simulink library "models"  (Simulink 7.2)
settings: Solver=ode45  SolverMode=SingleTasking  StartTime=0.0  StopTime=10.0  RelTol=1e-3
undefined symbols (not defined in the file or in its folder): actuator_T2_lib, aero, Aero, aero_lib, aftfuel, aftfuel_pos, Am, atmos, b, bias, Bm, Cbar, cg_pos0, cg_shift_gear, constants, DamageModels, Ed_trim_IC, engl_ang, engl_pos, engr_ang, engr_pos, fwdfuel, fwdfuel_pos, GTM_T2, hd_trim_IC, in_tadapton_forced, Inertia0, Inertia_shift_gear, latlonh_IC, MACH_U_nom_IC, Nd_trim_IC, pqr_trim_IC, quat_trim_IC, ref_cg, S, SENSOR, SERVO, symmetric_aero_on, trac_params, use_wind_meas_sim, vehicle_params, w0, xm0
libraries: simulink_need_slupdate x56, models x11, aeroutilslib x6, utility_lib x5, GTM_aerolib x4, model_lib x4, Polyval_lib x3, simulink x2, enginelib x2, engine_T2_lib x1
(part 1 of 4)
settings Model: Creator=E183308  LastModifiedBy=E183308

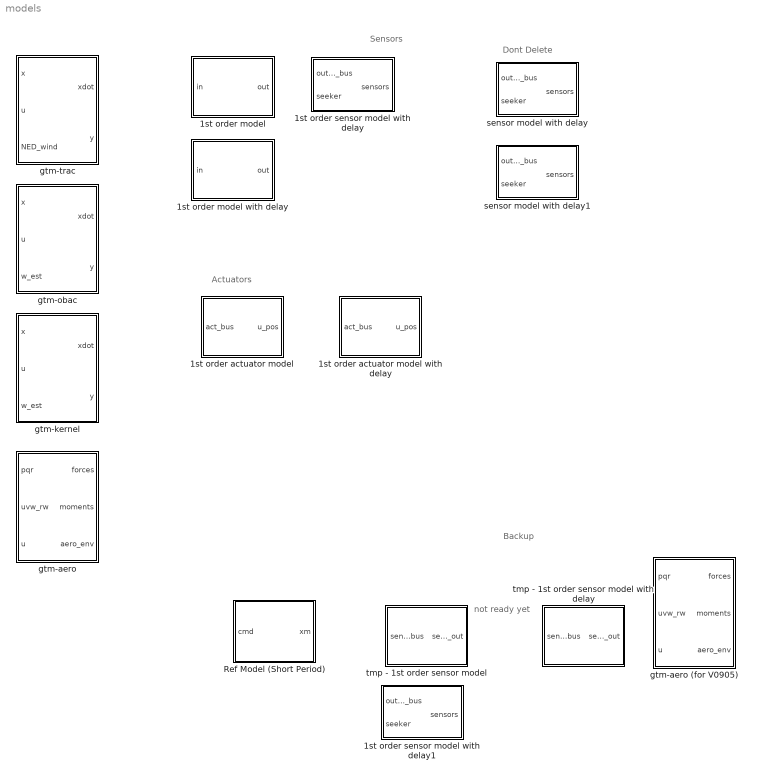
== system models ==
  note: Backup
  note: not ready yet
  note: Actuators
  note: Sensors
  note: Dont Delete
  1st order actuator model : Subsystem
  1st order actuator model with delay : Subsystem
  1st order model : Subsystem  mask{sens_idx=0}
      mask prompts: sens_idx "Indices"
  1st order model with delay : Subsystem  mask{sens_idx=0}
      mask prompts: sens_idx "Indices"
  1st order sensor model with delay : Subsystem
  1st order sensor model with delay1 : Subsystem
  Ref Model (Short Period) : Subsystem
  gtm-aero : Subsystem  mask{aero_params=aero}
      mask prompts: aero_params "aero params"
      mask init:
      | paramnames = fieldnames(aero_params);
      | for i=1:length(paramnames)
      | 	eval([paramnames{i} '= aero_params.' paramnames{i} ';']);
      | end
  gtm-aero (for V0905) : Subsystem  mask{aero_params=aero}
      mask prompts: aero_params "aero params"
      mask init:
      | paramnames = fieldnames(aero_params);
      | for i=1:length(paramnames)
      | 	eval([paramnames{i} '= aero_params.' paramnames{i} ';']);
      | end
  gtm-kernel : Subsystem  mask{vehicle_params=vehicle_params}
      mask prompts: vehicle_params "vehicle params"
      mask init:
      | paramnames = fieldnames(vehicle_params);
      | for i=1:length(paramnames)
      | 	eval([paramnames{i} '= vehicle_params.' paramnames{i} ';']);
      | end
  gtm-obac : Subsystem
  gtm-trac : Subsystem  mask{vehicle_params=trac_params}
      mask prompts: vehicle_params "vehicle params"
  sensor model with delay : Subsystem
  sensor model with delay1 : Subsystem
  tmp - 1st order sensor model : Subsystem
  tmp - 1st order sensor model with delay : Subsystem

== system models/1st order actuator model ==
  note: VARIABLE RATE LIMIT SERVO MODEL
      | (1st order)
  act_bus : Inport  OutDataType=sfix(16)  OutScaling=2^0
  Bus Selector1 : BusSelector  OutputSignals=effector_limits.u_ulim,effector_limits.u_llim,effector_limits.u_urlim,effector_limits.u_lrlim,u_cmd
  Enforce lower limit : MinMax  Function=max  Inputs=2  OutDataType=sfix(16)  OutScaling=2^-10  OutDataTypeStr=Inherit: Inherit via back propagation  ZeroCross=off
  Enforce lower limit1 : MinMax  Function=max  Inputs=2  OutDataType=sfix(16)  OutScaling=2^-10  OutDataTypeStr=Inherit: Inherit via back propagation  ZeroCross=off
  Enforce upper limit : MinMax  Inputs=2  OutDataType=sfix(16)  OutScaling=2^-10  OutDataTypeStr=Inherit: Inherit via back propagation  ZeroCross=off
  Enforce upper limit1 : MinMax  Inputs=2  OutDataType=sfix(16)  OutScaling=2^-10  OutDataTypeStr=Inherit: Inherit via back propagation  ZeroCross=off
  Sum : Sum  Inputs=|+-  OutDataType=sfix(16)  OutScaling=2^0  SaturateOnIntegerOverflow=on  InputSameDT=on  OutDataTypeStr=Inherit: Same as first input
  Sum1 : Sum  Inputs=|++  OutDataType=sfix(16)  OutScaling=2^0  SaturateOnIntegerOverflow=on  InputSameDT=on  OutDataTypeStr=Inherit: Same as first input
  Sum2 : Sum  Orientation=left  Inputs=-+|  OutDataType=sfix(16)  OutScaling=2^0  SaturateOnIntegerOverflow=on  InputSameDT=on  OutDataTypeStr=Inherit: Same as first input
  W : Gain  Gain=SERVO.w  ParameterDataType=sfix(16)  ParameterScaling=2^0  OutDataType=sfix(16)  OutScaling=2^0  SaturateOnIntegerOverflow=on  OutDataTypeStr=Inherit: Same as input  ParamDataTypeStr=Inherit: Same as input
  anti-windup gain : Gain  Orientation=left  Gain=SERVO.pos_Kaw  ParameterDataType=sfix(16)  ParameterScaling=2^0  OutDataType=sfix(16)  OutScaling=2^0
  pos integrator : Integrator  InitialCondition=SERVO.x0
  u_pos : Outport  OutDataType=sfix(16)  OutScaling=2^0
  wires:
  Bus Selector1/4 -> Enforce lower limit1/1  "<u_lrlim>"
  Bus Selector1/1 -> Enforce upper limit/1  "<u_ulim>"
  act_bus/1 -> Bus Selector1/1
  Enforce upper limit/1 -> Sum2/2, Sum/2, u_pos/1
  Enforce lower limit/1 -> Enforce upper limit/2
  pos integrator/1 -> Sum2/1, Enforce lower limit/2
  Sum2/1 -> anti-windup gain/1
  anti-windup gain/1 -> Sum1/2
  Sum1/1 -> pos integrator/1
  Sum/1 -> W/1
  Bus Selector1/5 -> Sum/1  "<u_cmd>"
  Bus Selector1/2 -> Enforce lower limit/1  "<u_llim>"
  Bus Selector1/3 -> Enforce upper limit1/1  "<u_urlim>"
  W/1 -> Enforce lower limit1/2
  Enforce lower limit1/1 -> Enforce upper limit1/2
  Enforce upper limit1/1 -> Sum1/1

== system models/1st order actuator model with delay ==
  note: VARIABLE RATE LIMIT SERVO MODEL
      | (1st order with delay)
  act_bus : Inport  OutDataType=sfix(16)  OutScaling=2^0
  1st order actuator model : models/1st order actuator model  SystemSampleTime=-1
  Transport Delay : TransportDelay  DelayTime=SERVO.delay  InitialOutput=SERVO.x0
  u_pos : Outport  OutDataType=sfix(16)  OutScaling=2^0
  wires:
  act_bus/1 -> 1st order actuator model/1
  1st order actuator model/1 -> Transport Delay/1
  Transport Delay/1 -> u_pos/1

== system models/1st order model ==
  note: 1st ORDER LIMIT MODEL
  in : Inport  OutDataType=sfix(16)  OutScaling=2^0
  Constant : Constant  Value=SENSOR.ulim(sens_idx)  OutDataType=sfix(16)  OutScaling=2^0
  Constant1 : Constant  Value=SENSOR.llim(sens_idx)  OutDataType=sfix(16)  OutScaling=2^0
  Enforce lower limit : MinMax  Function=max  Inputs=2  OutDataType=sfix(16)  OutScaling=2^-10  OutDataTypeStr=Inherit: Inherit via back propagation  ZeroCross=off
  Enforce upper limit : MinMax  Inputs=2  OutDataType=sfix(16)  OutScaling=2^-10  OutDataTypeStr=Inherit: Inherit via back propagation  ZeroCross=off
  Sum : Sum  Inputs=|+-  OutDataType=sfix(16)  OutScaling=2^0  SaturateOnIntegerOverflow=on  InputSameDT=on  OutDataTypeStr=Inherit: Same as first input
  W : Gain  Gain=SENSOR.w(sens_idx)  ParameterDataType=sfix(16)  ParameterScaling=2^0  OutDataType=sfix(16)  OutScaling=2^0  SaturateOnIntegerOverflow=on  OutDataTypeStr=Inherit: Same as input  ParamDataTypeStr=Inherit: Same as input
  integrator : Integrator  InitialCondition=SENSOR.x0(sens_idx)
  out : Outport  OutDataType=sfix(16)  OutScaling=2^0
  wires:
  Constant1/1 -> Enforce lower limit/1
  Sum/1 -> W/1
  integrator/1 -> Enforce lower limit/2
  Enforce lower limit/1 -> Enforce upper limit/2
  Enforce upper limit/1 -> out/1, Sum/2
  Constant/1 -> Enforce upper limit/1
  W/1 -> integrator/1
  in/1 -> Sum/1

== system models/1st order model with delay ==
  note: 1st ORDER LIMIT MODEL WITH DELAY
  in : Inport  OutDataType=sfix(16)  OutScaling=2^0
  Constant : Constant  Value=SENSOR.ulim(sens_idx)  OutDataType=sfix(16)  OutScaling=2^0
  Constant1 : Constant  Value=SENSOR.llim(sens_idx)  OutDataType=sfix(16)  OutScaling=2^0
  Enforce lower limit : MinMax  Function=max  Inputs=2  OutDataType=sfix(16)  OutScaling=2^-10  OutDataTypeStr=Inherit: Inherit via back propagation  ZeroCross=off
  Enforce upper limit : MinMax  Inputs=2  OutDataType=sfix(16)  OutScaling=2^-10  OutDataTypeStr=Inherit: Inherit via back propagation  ZeroCross=off
  Sum : Sum  Inputs=|+-  OutDataType=sfix(16)  OutScaling=2^0  SaturateOnIntegerOverflow=on  InputSameDT=on  OutDataTypeStr=Inherit: Same as first input
  W : Gain  Gain=SENSOR.w(sens_idx)  ParameterDataType=sfix(16)  ParameterScaling=2^0  OutDataType=sfix(16)  OutScaling=2^0  SaturateOnIntegerOverflow=on  OutDataTypeStr=Inherit: Same as input  ParamDataTypeStr=Inherit: Same as input
  delay : TransportDelay  DelayTime=SENSOR.delay  InitialOutput=SENSOR.x0(sens_idx)
  integrator : Integrator  InitialCondition=SENSOR.x0(sens_idx)
  out : Outport  OutDataType=sfix(16)  OutScaling=2^0
  wires:
  in/1 -> Sum/1
  W/1 -> integrator/1
  Constant/1 -> Enforce upper limit/1
  Enforce upper limit/1 -> Sum/2, delay/1
  Enforce lower limit/1 -> Enforce upper limit/2
  integrator/1 -> Enforce lower limit/2
  Sum/1 -> W/1
  Constant1/1 -> Enforce lower limit/1
  delay/1 -> out/1

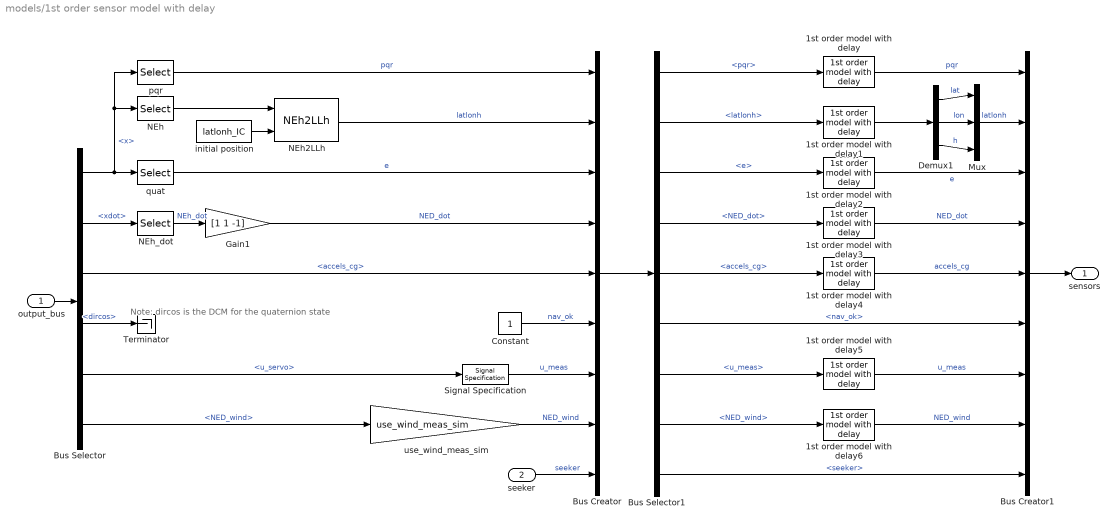
== system models/1st order sensor model with delay ==
  note: Note: dircos is the DCM
      | for the quaternion state
  output_bus : Inport  OutDataType=sfix(16)  OutScaling=2^0
  seeker : Inport  Port=2  OutDataType=sfix(16)  OutScaling=2^0
  1st order model with delay : models/1st order model with delay  SystemSampleTime=-1  sens_idx=SENSOR.pqr_idx
  1st order model with delay1 : models/1st order model with delay  SystemSampleTime=-1  sens_idx=SENSOR.latlonh_idx
  1st order model with delay2 : models/1st order model with delay  SystemSampleTime=-1  sens_idx=SENSOR.quat_idx
  1st order model with delay3 : models/1st order model with delay  SystemSampleTime=-1  sens_idx=SENSOR.NEDdot_idx
  1st order model with delay4 : models/1st order model with delay  SystemSampleTime=-1  sens_idx=SENSOR.accels_cg_idx
  1st order model with delay5 : models/1st order model with delay  SystemSampleTime=-1  sens_idx=SENSOR.umeas_idx
  1st order model with delay6 : models/1st order model with delay  SystemSampleTime=-1  sens_idx=SENSOR.NED_wind_idx
  Bus Creator : BusCreator  Inputs=9
  Bus Creator1 : BusCreator  Inputs=9
  Bus Selector : BusSelector  OutputSignals=x,xdot,y.accels_cg,y.dircos,u_servo,NED_wind
  Bus Selector1 : BusSelector  OutputSignals=pqr,latlonh,e,NED_dot,accels_cg,nav_ok,u_meas,NED_wind,seeker
  Constant : Constant  OutDataType=sfix(16)  OutScaling=2^0
  Demux1 : Demux  Outputs=3
  Gain1 : Gain  Gain=[1 1 -1]  ParameterDataType=sfix(16)  ParameterScaling=2^0  OutDataType=sfix(16)  OutScaling=2^0  SaturateOnIntegerOverflow=on  OutDataTypeStr=Inherit: Same as input  ParamDataTypeStr=Inherit: Same as input
  Mux : Mux  Inputs=3
  NEh : Selector  InputPortWidth=MACH.num_x  IndexOptions=Index vector (dialog)  Indices=MACH.NEh_idx  OutputSizes=1
  NEh2LLh : utility_lib/NEh2LLh  SystemSampleTime=-1
  NEh_dot : Selector  InputPortWidth=MACH.num_x  IndexOptions=Index vector (dialog)  Indices=MACH.NEh_idx  OutputSizes=1
  Signal Specification : SignalSpecification  OutDataType=sfix(16)  OutScaling=2^0
  Terminator : Terminator
  initial position : Constant  Value=latlonh_IC  OutDataType=sfix(16)  OutScaling=2^0
  pqr : Selector  InputPortWidth=MACH.num_x  IndexOptions=Index vector (dialog)  Indices=MACH.pqr_idx  OutputSizes=1
  quat : Selector  InputPortWidth=MACH.num_x  IndexOptions=Index vector (dialog)  Indices=MACH.quat_idx  OutputSizes=1
  use_wind_meas_sim : Gain  Gain=use_wind_meas_sim  ParameterDataType=sfix(16)  ParameterScaling=2^0  OutDataType=sfix(16)  OutScaling=2^0  SaturateOnIntegerOverflow=on  OutDataTypeStr=Inherit: Same as input  ParamDataTypeStr=Inherit: Same as input
  sensors : Outport  OutDataType=sfix(16)  OutScaling=2^0
  wires:
  1st order model with delay4/1 -> Bus Creator1/5  "accels_cg"
  1st order model with delay3/1 -> Bus Creator1/4  "NED_dot"
  1st order model with delay2/1 -> Bus Creator1/3  "e"
  1st order model with delay1/1 -> Demux1/1
  1st order model with delay6/1 -> Bus Creator1/8  "NED_wind"
  Bus Selector1/8 -> 1st order model with delay6/1  "<NED_wind>"
  1st order model with delay5/1 -> Bus Creator1/7  "u_meas"
  Bus Selector1/7 -> 1st order model with delay5/1  "<u_meas>"
  Bus Selector1/5 -> 1st order model with delay4/1  "<accels_cg>"
  Bus Selector1/4 -> 1st order model with delay3/1  "<NED_dot>"
  Bus Selector1/3 -> 1st order model with delay2/1  "<e>"
  Bus Selector1/2 -> 1st order model with delay1/1  "<latlonh>"
  Bus Selector1/1 -> 1st order model with delay/1  "<pqr>"
  Bus Selector1/9 -> Bus Creator1/9  "<seeker>"
  1st order model with delay/1 -> Bus Creator1/1  "pqr"
  Bus Creator/1 -> Bus Selector1/1
  Mux/1 -> Bus Creator1/2  "latlonh"
  Demux1/3 -> Mux/3  "h"
  Demux1/2 -> Mux/2  "lon"
  Demux1/1 -> Mux/1  "lat"
  Bus Creator1/1 -> sensors/1
  Signal Specification/1 -> Bus Creator/7  "u_meas"
  Bus Selector/5 -> Signal Specification/1  "<u_servo>"
  use_wind_meas_sim/1 -> Bus Creator/8  "NED_wind"
  Gain1/1 -> Bus Creator/4  "NED_dot"
  NEh2LLh/1 -> Bus Creator/2  "latlonh"
  pqr/1 -> Bus Creator/1  "pqr"
  NEh_dot/1 -> Gain1/1  "NEh_dot"
  Bus Selector/2 -> NEh_dot/1  "<xdot>"
  quat/1 -> Bus Creator/3  "e"
  initial position/1 -> NEh2LLh/2
  Constant/1 -> Bus Creator/6  "nav_ok"
  NEh/1 -> NEh2LLh/1
  output_bus/1 -> Bus Selector/1
  Bus Selector/6 -> use_wind_meas_sim/1  "<NED_wind>"
  seeker/1 -> Bus Creator/9  "seeker"
  Bus Selector/1 -> quat/1, NEh/1, pqr/1  "<x>"
  Bus Selector/3 -> Bus Creator/5  "<accels_cg>"
  Bus Selector/4 -> Terminator/1  "<dircos>"
  Bus Selector1/6 -> Bus Creator1/6  "<nav_ok>"

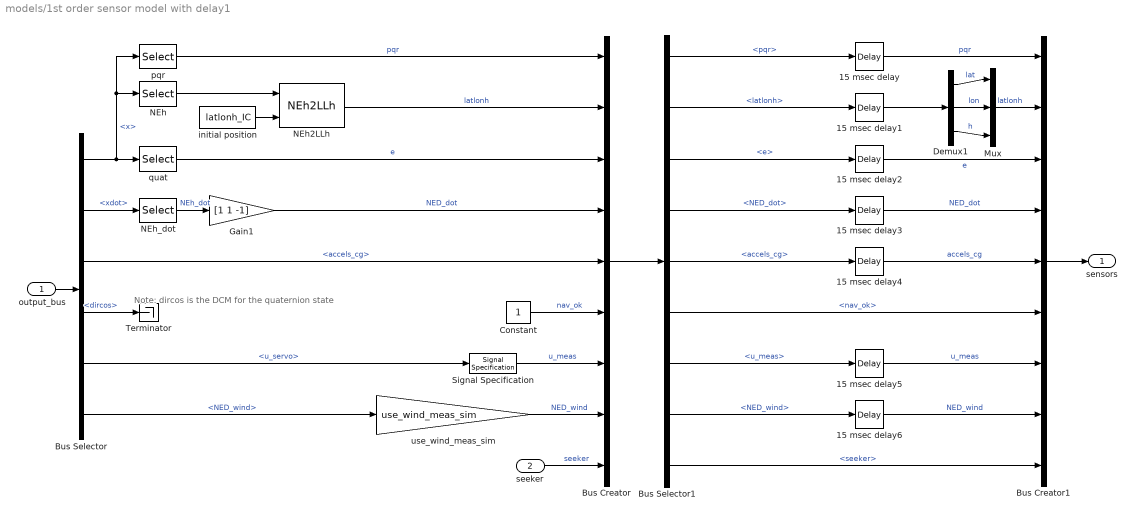
== system models/1st order sensor model with delay1 ==
  note: Note: dircos is the DCM
      | for the quaternion state
  output_bus : Inport  OutDataType=sfix(16)  OutScaling=2^0
  seeker : Inport  Port=2  OutDataType=sfix(16)  OutScaling=2^0
  15 msec delay : TransportDelay  DelayTime=15e-3  InitialOutput=pqr_trim_IC
  15 msec delay1 : TransportDelay  DelayTime=15e-3  InitialOutput=latlonh_IC
  15 msec delay2 : TransportDelay  DelayTime=15e-3  InitialOutput=quat_trim_IC
  15 msec delay3 : TransportDelay  DelayTime=15e-3  InitialOutput=[Nd_trim_IC Ed_trim_IC -hd_trim_IC]
  15 msec delay4 : TransportDelay  DelayTime=15e-3  InitialOutput=[0 0 0]'
  15 msec delay5 : TransportDelay  DelayTime=15e-3  InitialOutput=MACH_U_nom_IC
  15 msec delay6 : TransportDelay  DelayTime=15e-3  InitialOutput=[0 0 0]'
  Bus Creator : BusCreator  Inputs=9
  Bus Creator1 : BusCreator  Inputs=9
  Bus Selector : BusSelector  OutputSignals=x,xdot,y.accels_cg,y.dircos,u_servo,NED_wind
  Bus Selector1 : BusSelector  OutputSignals=pqr,latlonh,e,NED_dot,accels_cg,nav_ok,u_meas,NED_wind,seeker
  Constant : Constant  OutDataType=sfix(16)  OutScaling=2^0
  Demux1 : Demux  Outputs=3
  Gain1 : Gain  Gain=[1 1 -1]  ParameterDataType=sfix(16)  ParameterScaling=2^0  OutDataType=sfix(16)  OutScaling=2^0  SaturateOnIntegerOverflow=on  OutDataTypeStr=Inherit: Same as input  ParamDataTypeStr=Inherit: Same as input
  Mux : Mux  Inputs=3
  NEh : Selector  InputPortWidth=MACH.num_x  IndexOptions=Index vector (dialog)  Indices=MACH.NEh_idx  OutputSizes=1
  NEh2LLh : utility_lib/NEh2LLh  SystemSampleTime=-1
  NEh_dot : Selector  InputPortWidth=MACH.num_x  IndexOptions=Index vector (dialog)  Indices=MACH.NEh_idx  OutputSizes=1
  Signal Specification : SignalSpecification  OutDataType=sfix(16)  OutScaling=2^0
  Terminator : Terminator
  initial position : Constant  Value=latlonh_IC  OutDataType=sfix(16)  OutScaling=2^0
  pqr : Selector  InputPortWidth=MACH.num_x  IndexOptions=Index vector (dialog)  Indices=MACH.pqr_idx  OutputSizes=1
  quat : Selector  InputPortWidth=MACH.num_x  IndexOptions=Index vector (dialog)  Indices=MACH.quat_idx  OutputSizes=1
  use_wind_meas_sim : Gain  Gain=use_wind_meas_sim  ParameterDataType=sfix(16)  ParameterScaling=2^0  OutDataType=sfix(16)  OutScaling=2^0  SaturateOnIntegerOverflow=on  OutDataTypeStr=Inherit: Same as input  ParamDataTypeStr=Inherit: Same as input
  sensors : Outport  OutDataType=sfix(16)  OutScaling=2^0
  wires:
  Bus Selector1/6 -> Bus Creator1/6  "<nav_ok>"
  Bus Selector/4 -> Terminator/1  "<dircos>"
  Bus Selector/3 -> Bus Creator/5  "<accels_cg>"
  Bus Selector/1 -> pqr/1, NEh/1, quat/1  "<x>"
  seeker/1 -> Bus Creator/9  "seeker"
  Bus Selector/6 -> use_wind_meas_sim/1  "<NED_wind>"
  output_bus/1 -> Bus Selector/1
  NEh/1 -> NEh2LLh/1
  Constant/1 -> Bus Creator/6  "nav_ok"
  initial position/1 -> NEh2LLh/2
  quat/1 -> Bus Creator/3  "e"
  Bus Selector/2 -> NEh_dot/1  "<xdot>"
  NEh_dot/1 -> Gain1/1  "NEh_dot"
  pqr/1 -> Bus Creator/1  "pqr"
  NEh2LLh/1 -> Bus Creator/2  "latlonh"
  Gain1/1 -> Bus Creator/4  "NED_dot"
  use_wind_meas_sim/1 -> Bus Creator/8  "NED_wind"
  Bus Selector/5 -> Signal Specification/1  "<u_servo>"
  Signal Specification/1 -> Bus Creator/7  "u_meas"
  Bus Creator1/1 -> sensors/1
  Demux1/1 -> Mux/1  "lat"
  Demux1/2 -> Mux/2  "lon"
  Demux1/3 -> Mux/3  "h"
  Mux/1 -> Bus Creator1/2  "latlonh"
  Bus Creator/1 -> Bus Selector1/1
  15 msec delay/1 -> Bus Creator1/1  "pqr"
  Bus Selector1/9 -> Bus Creator1/9  "<seeker>"
  Bus Selector1/1 -> 15 msec delay/1  "<pqr>"
  Bus Selector1/2 -> 15 msec delay1/1  "<latlonh>"
  Bus Selector1/3 -> 15 msec delay2/1  "<e>"
  Bus Selector1/4 -> 15 msec delay3/1  "<NED_dot>"
  Bus Selector1/5 -> 15 msec delay4/1  "<accels_cg>"
  Bus Selector1/7 -> 15 msec delay5/1  "<u_meas>"
  15 msec delay5/1 -> Bus Creator1/7  "u_meas"
  Bus Selector1/8 -> 15 msec delay6/1  "<NED_wind>"
  15 msec delay6/1 -> Bus Creator1/8  "NED_wind"
  15 msec delay1/1 -> Demux1/1
  15 msec delay2/1 -> Bus Creator1/3  "e"
  15 msec delay3/1 -> Bus Creator1/4  "NED_dot"
  15 msec delay4/1 -> Bus Creator1/5  "accels_cg"

== system models/Ref Model (Short Period) ==
  cmd : Inport  OutDataType=sfix(16)  OutScaling=2^0
  Am : Gain  Orientation=left  Gain=Am  Multiplication=Matrix(K*u)  ParameterDataType=sfix(16)  ParameterScaling=2^0  OutDataType=sfix(16)  OutScaling=2^0
  Bm : Gain  Gain=Bm  Multiplication=Matrix(K*u)  ParameterDataType=sfix(16)  ParameterScaling=2^0  OutDataType=sfix(16)  OutScaling=2^0
  Clock : Clock
      settings: Decimation=10
  Compare To Constant : simulink/Logic and Bit Operations/Compare To Constant  SystemSampleTime=-1  relop=>=  const=in_tadapton_forced  LogicOutDataTypeMode=boolean  ZeroCross=off
  Constant : Constant  Value=[0 0 0]  OutDataType=sfix(16)  OutScaling=2^0
  Constant1 : Constant  Value="[0.0215    0.0052    0.0041]"  OutDataType=sfix(16)  OutScaling=2^0
  Gain : Gain  Gain=180/pi  ParameterDataType=sfix(16)  ParameterScaling=2^0  OutDataType=sfix(16)  OutScaling=2^0
  Gain1 : Gain  Gain=180/pi  ParameterDataType=sfix(16)  ParameterScaling=2^0  OutDataType=sfix(16)  OutScaling=2^0
  Gain2 : Gain  Gain=180/pi  ParameterDataType=sfix(16)  ParameterScaling=2^0  OutDataType=sfix(16)  OutScaling=2^0
  Integrator : Integrator  ExternalReset=rising  InitialConditionSource=external  InitialCondition=xm0
  Sum2 : Sum  Inputs=|++  OutDataType=sfix(16)  OutScaling=2^0
  Switch : Switch  Threshold=in_tadapton_forced  OutDataType=sfix(16)  OutScaling=2^0
  alpha (deg) : Scope
      settings: SaveName=ScopeData22
  alpham : Selector  InputPortWidth=3  IndexOptions=Index vector (dialog)  Indices=3  OutputSizes=1
  qcmd (deg/s) : Scope
      settings: YMin=-1  YMax=1  SaveName=ScopeData5
  qm : Selector  InputPortWidth=3  IndexOptions=Index vector (dialog)  Indices=2  OutputSizes=1
  qm (deg/s) : Scope
      settings: SaveName=ScopeData3
  qm1 : Selector  InputPortWidth=3  IndexOptions=Index vector (dialog)  Indices=1  OutputSizes=1
  xcm : Scope
      settings: SaveName=ScopeData9
  xm : Outport  OutDataType=sfix(16)  OutScaling=2^0
  wires:
  cmd/1 -> Bm/1, Gain2/1
  Integrator/1 -> Am/1, xm/1, qm1/1, qm/1, alpham/1
  Am/1 -> Sum2/2
  Sum2/1 -> Integrator/1
  Bm/1 -> Sum2/1
  qm/1 -> Gain/1
  alpham/1 -> Gain1/1
  Gain/1 -> qm (deg/s)/1
  Gain1/1 -> alpha (deg)/1
  Gain2/1 -> qcmd (deg/s)/1
  qm1/1 -> xcm/1
  Switch/1 -> Integrator/3
  Constant1/1 -> Switch/1
  Constant/1 -> Switch/3
  Clock/1 -> Switch/2, Compare To Constant/1
  Compare To Constant/1 -> Integrator/2

== system models/gtm-aero ==
  pqr : Inport  OutDataType=sfix(16)  OutScaling=2^0
  uvw_rw : Inport  Port=2  OutDataType=sfix(16)  OutScaling=2^0
  u : Inport  Port=3  OutDataType=sfix(16)  OutScaling=2^0
  A/C parameters : Subsystem  AncestorBlock=acparams_lib/A//C parameters
  Aero_GTM_T2 : Subsystem  AncestorBlock=aero_lib/GTM_T2
  AuxVars_Reduced : Subsystem
  Bus Selector4 : BusSelector  OutputSignals=atmos_env.sos,atmos_env.rho,atmos_env.h,atmos_env.P,atmos_env.T
  Demux : Demux  Outputs=[3 3]
  GTM_T2_MACH : engine_T2_lib/GTM_T2_MACH  SystemSampleTime=-1
  Goto Tag Visibility : GotoTagVisibility  GotoTag=AC_Params
  Sum : Sum  OutDataType=sfix(16)  OutScaling=2^0
  Terminator : Terminator
  aero surf ganging : Subsystem
  get aero environment : model_lib/get aero environment  SystemSampleTime=-1
  forces : Outport  OutDataType=sfix(16)  OutScaling=2^0
  moments : Outport  Port=2  OutDataType=sfix(16)  OutScaling=2^0
  aero_env : Outport  Port=3  OutDataType=sfix(16)  OutScaling=2^0
  tag scope: AC_Params=scoped
  wires:
  u/1 -> aero surf ganging/1(u)
  uvw_rw/1 -> get aero environment/1
  pqr/1 -> AuxVars_Reduced/1(pqr)
  get aero environment/1 -> aero_env/1, AuxVars_Reduced/2(aero_env)
  Bus Selector4/1 -> get aero environment/2  "<sos>"
  Bus Selector4/2 -> get aero environment/3  "<rho>"
  Bus Selector4/3 -> get aero environment/4  "<h>"
  Bus Selector4/4 -> AuxVars_Reduced/3(P)  "<P>"
  Bus Selector4/5 -> AuxVars_Reduced/4(T)  "<T>"
  aero surf ganging/1(cmds) -> Aero_GTM_T2/1(Surfaces), GTM_T2_MACH/1, A/C parameters/2(Surfaces)
  AuxVars_Reduced/1(AuxVars) -> Aero_GTM_T2/2(AuxVars), GTM_T2_MACH/2
  AuxVars_Reduced/2(State) -> Aero_GTM_T2/3(State), GTM_T2_MACH/3
  GTM_T2_MACH/1 -> A/C parameters/1(Engines), Aero_GTM_T2/4(Engines)
  GTM_T2_MACH/2 -> Sum/1
  Aero_GTM_T2/1(FM) -> Sum/2
  Aero_GTM_T2/2(Aero) -> Terminator/1
  Sum/1 -> Demux/1
  Demux/1 -> forces/1
  Demux/2 -> moments/1
  A/C parameters/1(AC_parameters) -> [AC_Params], GTM_T2_MACH/4
  [scoped_bus] -> Bus Selector4/1

== system models/gtm-aero (for V0905) ==
  pqr : Inport  OutDataType=sfix(16)  OutScaling=2^0
  uvw_rw : Inport  Port=2  OutDataType=sfix(16)  OutScaling=2^0
  u : Inport  Port=3  OutDataType=sfix(16)  OutScaling=2^0
  A/C parameters : Subsystem  AncestorBlock=acparams_lib/A//C parameters
  Aero_GTM_T2 : Subsystem  AncestorBlock=aero_lib/GTM_T2
  AuxVars_Reduced : Subsystem
  Bus Selector4 : BusSelector  OutputSignals=atmos_env.sos,atmos_env.rho,atmos_env.h,atmos_env.P,atmos_env.T
  Demux : Demux  Outputs=[3 3]
  Eng_GTM_T2 : Subsystem  AncestorBlock=engine_T2_lib/GTM_T2
  Goto Tag Visibility : GotoTagVisibility  GotoTag=AC_Params
  Sum : Sum  OutDataType=sfix(16)  OutScaling=2^0
  Terminator : Terminator
  aero surf ganging : Subsystem
  get aero environment : model_lib/get aero environment  SystemSampleTime=-1
  forces : Outport  OutDataType=sfix(16)  OutScaling=2^0
  moments : Outport  Port=2  OutDataType=sfix(16)  OutScaling=2^0
  aero_env : Outport  Port=3  OutDataType=sfix(16)  OutScaling=2^0
  tag scope: AC_Params=scoped
  wires:
  [scoped_bus] -> Bus Selector4/1
  A/C parameters/1(AC_parameters) -> Eng_GTM_T2/4(AC_Params), [AC_Params]
  Demux/2 -> moments/1
  Demux/1 -> forces/1
  Sum/1 -> Demux/1
  Aero_GTM_T2/2(Aero) -> Terminator/1
  Aero_GTM_T2/1(FM) -> Sum/2
  Eng_GTM_T2/2(FM) -> Sum/1
  Eng_GTM_T2/1(Engines) -> Aero_GTM_T2/4(Engines), A/C parameters/1(Engines)
  AuxVars_Reduced/2(State) -> Eng_GTM_T2/3(State), Aero_GTM_T2/3(State)
  AuxVars_Reduced/1(AuxVars) -> Eng_GTM_T2/2(AuxVars), Aero_GTM_T2/2(AuxVars)
  aero surf ganging/1(cmds) -> A/C parameters/2(Surfaces), Eng_GTM_T2/1(cmds), Aero_GTM_T2/1(Surfaces)
  Bus Selector4/5 -> AuxVars_Reduced/4(T)  "<T>"
  Bus Selector4/4 -> AuxVars_Reduced/3(P)  "<P>"
  Bus Selector4/3 -> get aero environment/4  "<h>"
  Bus Selector4/2 -> get aero environment/3  "<rho>"
  Bus Selector4/1 -> get aero environment/2  "<sos>"
  get aero environment/1 -> AuxVars_Reduced/2(aero_env), aero_env/1
  pqr/1 -> AuxVars_Reduced/1(pqr)
  uvw_rw/1 -> get aero environment/1
  u/1 -> aero surf ganging/1(u)

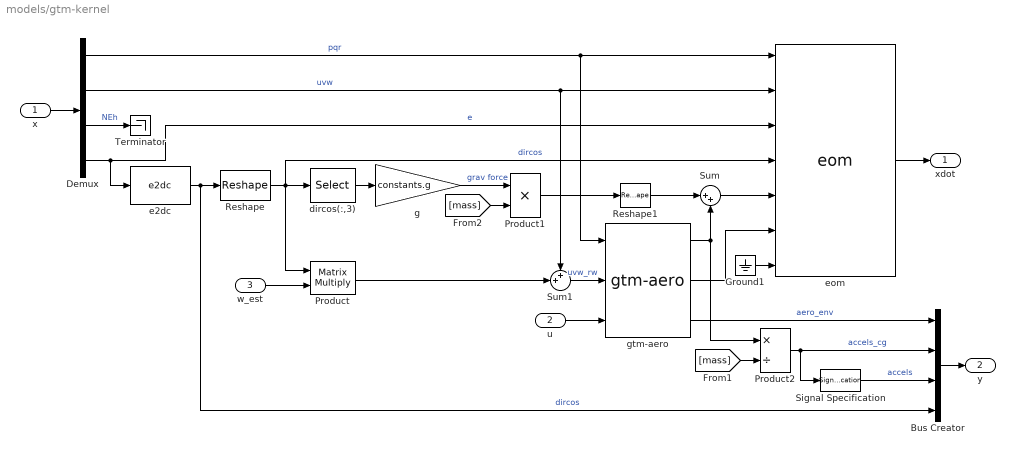
== system models/gtm-kernel ==
  x : Inport  OutDataType=sfix(16)  OutScaling=2^0
  u : Inport  Port=2  OutDataType=sfix(16)  OutScaling=2^0
  w_est : Inport  Port=3  OutDataType=sfix(16)  OutScaling=2^0
  Bus Creator : BusCreator
  Demux : Demux  Outputs=[3 3 3 4]
  Ground1 : Ground
  Product : Product  Multiplication=Matrix(*)  OutDataType=sfix(16)  OutScaling=2^0  SaturateOnIntegerOverflow=on  OutDataTypeStr=Inherit: Same as first input
  Product1 : Product  OutDataType=sfix(16)  OutScaling=2^0  RndMeth=Zero
  Product2 : Product  Inputs=*/  OutDataType=sfix(16)  OutScaling=2^0  RndMeth=Zero
  Reshape : Reshape  OutputDimensionality=Customize  OutputDimensions=[3,3]
  Reshape1 : Reshape
  Signal Specification : SignalSpecification  Dimensions=3  OutDataType=sfix(16)  OutScaling=2^0
  Sum : Sum  Inputs=|++  OutDataType=sfix(16)  OutScaling=2^0  SaturateOnIntegerOverflow=on
  Sum1 : Sum  Inputs=++|  OutDataType=sfix(16)  OutScaling=2^0  SaturateOnIntegerOverflow=on
  Terminator : Terminator
  dircos(:,3) : Selector  NumberOfDimensions=2  InputPortWidth=9  IndexOptions=Select all,Index vector (dialog)  Indices=-1,3  OutputSizes=1
  e2dc : utility_lib/e2dc  SystemSampleTime=-1
  eom : model_lib/eom  SystemSampleTime=-1
  g : Gain  Gain=constants.g  ParameterDataType=sfix(16)  ParameterScaling=2^0  OutDataType=sfix(16)  OutScaling=2^0  SaturateOnIntegerOverflow=on  OutDataTypeStr=Inherit: Same as input  ParamDataTypeStr=Inherit: Same as input
  gtm-aero : models/gtm-aero  SystemSampleTime=-1  aero_params=aero
  xdot : Outport  OutDataType=sfix(16)  OutScaling=2^0
  y : Outport  Port=2  OutDataType=sfix(16)  OutScaling=2^0
  wires:
  Ground1/1 -> eom/7
  Product1/1 -> Reshape1/1
  [mass] -> Product1/2
  g/1 -> Product1/1  "grav force"
  x/1 -> Demux/1
  Demux/1 -> eom/1, gtm-aero/1  "pqr"
  Demux/3 -> Terminator/1  "NEh"
  Demux/4 -> eom/3, e2dc/1  "e"
  Demux/2 -> eom/2, Sum1/1  "uvw"
  dircos(:,3)/1 -> g/1
  eom/1 -> xdot/1
  e2dc/1 -> Reshape/1, Bus Creator/4  "dircos"
  u/1 -> gtm-aero/3
  gtm-aero/1 -> Sum/2, Product2/1
  Sum1/1 -> gtm-aero/2  "uvw_rw"
  w_est/1 -> Product/2
  Product/1 -> Sum1/2
  Sum/1 -> eom/5
  Reshape/1 -> eom/4, dircos(:,3)/1, Product/1  "dircos"
  gtm-aero/2 -> eom/6
  gtm-aero/3 -> Bus Creator/1  "aero_env"
  Product2/1 -> Bus Creator/2, Signal Specification/1  "accels_cg"
  [mass] -> Product2/2
  Signal Specification/1 -> Bus Creator/3  "accels"
  Bus Creator/1 -> y/1
  Reshape1/1 -> Sum/1

== system models/gtm-obac ==
  x : Inport  OutDataType=sfix(16)  OutScaling=2^0
  u : Inport  Port=2  OutDataType=sfix(16)  OutScaling=2^0
  w_est : Inport  Port=3  OutDataType=sfix(16)  OutScaling=2^0
  gtm-kernel : models/gtm-kernel  SystemSampleTime=-1  vehicle_params=obac_params
  xdot : Outport  OutDataType=sfix(16)  OutScaling=2^0
  y : Outport  Port=2  OutDataType=sfix(16)  OutScaling=2^0
  wires:
  gtm-kernel/2 -> y/1
  gtm-kernel/1 -> xdot/1
  w_est/1 -> gtm-kernel/3
  u/1 -> gtm-kernel/2
  x/1 -> gtm-kernel/1

== system models/gtm-trac ==
  x : Inport  OutDataType=sfix(16)  OutScaling=2^0
  u : Inport  Port=2  OutDataType=sfix(16)  OutScaling=2^0
  NED_wind : Inport  Port=3  OutDataType=sfix(16)  OutScaling=2^0
  Bus Assignment : BusAssignment  AssignedSignals=accels
  Bus Selector : BusSelector  OutputSignals=accels_cg
  accel at sensor : model_lib/accel at sensor  SystemSampleTime=-1  vehicle_params=vehicle_params
  gtm-kernel : models/gtm-kernel  SystemSampleTime=-1  vehicle_params=vehicle_params
  xdot : Outport  OutDataType=sfix(16)  OutScaling=2^0
  y : Outport  Port=2  OutDataType=sfix(16)  OutScaling=2^0
  wires:
  Bus Assignment/1 -> y/1
  NED_wind/1 -> gtm-kernel/3
  x/1 -> accel at sensor/3, gtm-kernel/1
  u/1 -> gtm-kernel/2
  gtm-kernel/1 -> xdot/1, accel at sensor/1
  accel at sensor/1 -> Bus Assignment/2
  gtm-kernel/2 -> Bus Selector/1, Bus Assignment/1
  Bus Selector/1 -> accel at sensor/2  "<accels_cg>"

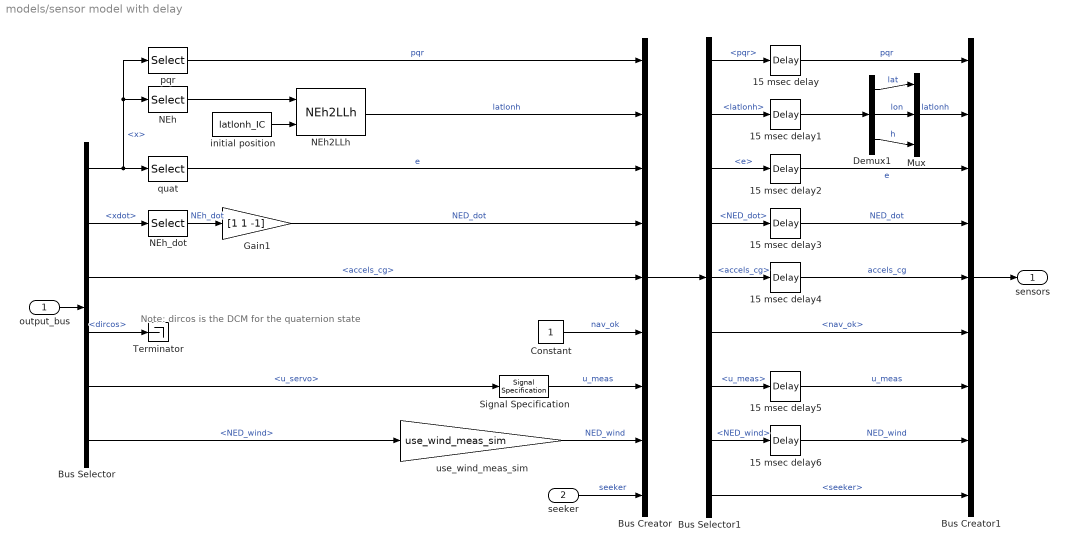
== system models/sensor model with delay ==
  note: Note: dircos is the DCM
      | for the quaternion state
  output_bus : Inport  OutDataType=sfix(16)  OutScaling=2^0
  seeker : Inport  Port=2  OutDataType=sfix(16)  OutScaling=2^0
  15 msec delay : TransportDelay  DelayTime=15e-3  InitialOutput=pqr_trim_IC
  15 msec delay1 : TransportDelay  DelayTime=15e-3  InitialOutput=latlonh_IC
  15 msec delay2 : TransportDelay  DelayTime=15e-3  InitialOutput=quat_trim_IC
  15 msec delay3 : TransportDelay  DelayTime=15e-3  InitialOutput=[Nd_trim_IC Ed_trim_IC -hd_trim_IC]
  15 msec delay4 : TransportDelay  DelayTime=15e-3  InitialOutput=[0 0 0]'
  15 msec delay5 : TransportDelay  DelayTime=15e-3  InitialOutput=MACH_U_nom_IC
  15 msec delay6 : TransportDelay  DelayTime=15e-3  InitialOutput=[0 0 0]
  Bus Creator : BusCreator  Inputs=9
  Bus Creator1 : BusCreator  Inputs=9
  Bus Selector : BusSelector  OutputSignals=x,xdot,y.accels_cg,y.dircos,u_servo,NED_wind
  Bus Selector1 : BusSelector  OutputSignals=pqr,latlonh,e,NED_dot,accels_cg,nav_ok,u_meas,NED_wind,seeker
  Constant : Constant  OutDataType=sfix(16)  OutScaling=2^0
  Demux1 : Demux  Outputs=3
  Gain1 : Gain  Gain=[1 1 -1]  ParameterDataType=sfix(16)  ParameterScaling=2^0  OutDataType=sfix(16)  OutScaling=2^0  SaturateOnIntegerOverflow=on  OutDataTypeStr=Inherit: Same as input  ParamDataTypeStr=Inherit: Same as input
  Mux : Mux  Inputs=3
  NEh : Selector  InputPortWidth=MACH.num_x  IndexOptions=Index vector (dialog)  Indices=MACH.NEh_idx  OutputSizes=1
  NEh2LLh : utility_lib/NEh2LLh  SystemSampleTime=-1
  NEh_dot : Selector  InputPortWidth=MACH.num_x  IndexOptions=Index vector (dialog)  Indices=MACH.NEh_idx  OutputSizes=1
  Signal Specification : SignalSpecification  OutDataType=sfix(16)  OutScaling=2^0
  Terminator : Terminator
  initial position : Constant  Value=latlonh_IC  OutDataType=sfix(16)  OutScaling=2^0
  pqr : Selector  InputPortWidth=MACH.num_x  IndexOptions=Index vector (dialog)  Indices=MACH.pqr_idx  OutputSizes=1
  quat : Selector  InputPortWidth=MACH.num_x  IndexOptions=Index vector (dialog)  Indices=MACH.quat_idx  OutputSizes=1
  use_wind_meas_sim : Gain  Gain=use_wind_meas_sim  ParameterDataType=sfix(16)  ParameterScaling=2^0  OutDataType=sfix(16)  OutScaling=2^0  SaturateOnIntegerOverflow=on  OutDataTypeStr=Inherit: Same as input  ParamDataTypeStr=Inherit: Same as input
  sensors : Outport  OutDataType=sfix(16)  OutScaling=2^0
  wires:
  Bus Selector/4 -> Terminator/1  "<dircos>"
  Bus Selector/3 -> Bus Creator/5  "<accels_cg>"
  Bus Selector/1 -> pqr/1, NEh/1, quat/1  "<x>"
  seeker/1 -> Bus Creator/9  "seeker"
  Bus Selector/6 -> use_wind_meas_sim/1  "<NED_wind>"
  output_bus/1 -> Bus Selector/1
  NEh/1 -> NEh2LLh/1
  Constant/1 -> Bus Creator/6  "nav_ok"
  initial position/1 -> NEh2LLh/2
  quat/1 -> Bus Creator/3  "e"
  Bus Selector/2 -> NEh_dot/1  "<xdot>"
  NEh_dot/1 -> Gain1/1  "NEh_dot"
  pqr/1 -> Bus Creator/1  "pqr"
  NEh2LLh/1 -> Bus Creator/2  "latlonh"
  Gain1/1 -> Bus Creator/4  "NED_dot"
  use_wind_meas_sim/1 -> Bus Creator/8  "NED_wind"
  Bus Selector/5 -> Signal Specification/1  "<u_servo>"
  Signal Specification/1 -> Bus Creator/7  "u_meas"
  Bus Creator1/1 -> sensors/1
  Demux1/1 -> Mux/1  "lat"
  Demux1/2 -> Mux/2  "lon"
  Demux1/3 -> Mux/3  "h"
  Mux/1 -> Bus Creator1/2  "latlonh"
  Bus Creator/1 -> Bus Selector1/1
  15 msec delay/1 -> Bus Creator1/1  "pqr"
  Bus Selector1/9 -> Bus Creator1/9  "<seeker>"
  Bus Selector1/1 -> 15 msec delay/1  "<pqr>"
  Bus Selector1/2 -> 15 msec delay1/1  "<latlonh>"
  Bus Selector1/3 -> 15 msec delay2/1  "<e>"
  Bus Selector1/4 -> 15 msec delay3/1  "<NED_dot>"
  Bus Selector1/5 -> 15 msec delay4/1  "<accels_cg>"
  Bus Selector1/6 -> Bus Creator1/6  "<nav_ok>"
  Bus Selector1/7 -> 15 msec delay5/1  "<u_meas>"
  15 msec delay5/1 -> Bus Creator1/7  "u_meas"
  Bus Selector1/8 -> 15 msec delay6/1  "<NED_wind>"
  15 msec delay6/1 -> Bus Creator1/8  "NED_wind"
  15 msec delay1/1 -> Demux1/1
  15 msec delay2/1 -> Bus Creator1/3  "e"
  15 msec delay3/1 -> Bus Creator1/4  "NED_dot"
  15 msec delay4/1 -> Bus Creator1/5  "accels_cg"

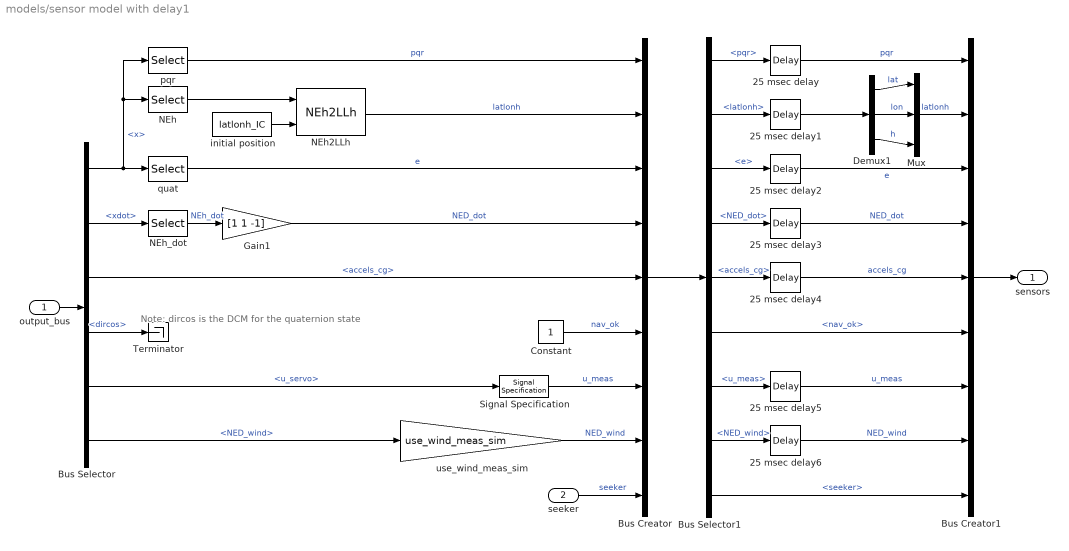
== system models/sensor model with delay1 ==
  note: Note: dircos is the DCM
      | for the quaternion state
  output_bus : Inport  OutDataType=sfix(16)  OutScaling=2^0
  seeker : Inport  Port=2  OutDataType=sfix(16)  OutScaling=2^0
  25 msec delay : TransportDelay  DelayTime=25e-3  InitialOutput=pqr_trim_IC
  25 msec delay1 : TransportDelay  DelayTime=25e-3  InitialOutput=latlonh_IC
  25 msec delay2 : TransportDelay  DelayTime=25e-3  InitialOutput=quat_trim_IC
  25 msec delay3 : TransportDelay  DelayTime=25e-3  InitialOutput=[Nd_trim_IC Ed_trim_IC -hd_trim_IC]
  25 msec delay4 : TransportDelay  DelayTime=25e-3  InitialOutput=[0 0 0]'
  25 msec delay5 : TransportDelay  DelayTime=25e-3  InitialOutput=MACH_U_nom_IC
  25 msec delay6 : TransportDelay  DelayTime=25e-3  InitialOutput=[0 0 0]
  Bus Creator : BusCreator  Inputs=9
  Bus Creator1 : BusCreator  Inputs=9
  Bus Selector : BusSelector  OutputSignals=x,xdot,y.accels_cg,y.dircos,u_servo,NED_wind
  Bus Selector1 : BusSelector  OutputSignals=pqr,latlonh,e,NED_dot,accels_cg,nav_ok,u_meas,NED_wind,seeker
  Constant : Constant  OutDataType=sfix(16)  OutScaling=2^0
  Demux1 : Demux  Outputs=3
  Gain1 : Gain  Gain=[1 1 -1]  ParameterDataType=sfix(16)  ParameterScaling=2^0  OutDataType=sfix(16)  OutScaling=2^0  SaturateOnIntegerOverflow=on  OutDataTypeStr=Inherit: Same as input  ParamDataTypeStr=Inherit: Same as input
  Mux : Mux  Inputs=3
  NEh : Selector  InputPortWidth=MACH.num_x  IndexOptions=Index vector (dialog)  Indices=MACH.NEh_idx  OutputSizes=1
  NEh2LLh : utility_lib/NEh2LLh  SystemSampleTime=-1
  NEh_dot : Selector  InputPortWidth=MACH.num_x  IndexOptions=Index vector (dialog)  Indices=MACH.NEh_idx  OutputSizes=1
  Signal Specification : SignalSpecification  OutDataType=sfix(16)  OutScaling=2^0
  Terminator : Terminator
  initial position : Constant  Value=latlonh_IC  OutDataType=sfix(16)  OutScaling=2^0
  pqr : Selector  InputPortWidth=MACH.num_x  IndexOptions=Index vector (dialog)  Indices=MACH.pqr_idx  OutputSizes=1
  quat : Selector  InputPortWidth=MACH.num_x  IndexOptions=Index vector (dialog)  Indices=MACH.quat_idx  OutputSizes=1
  use_wind_meas_sim : Gain  Gain=use_wind_meas_sim  ParameterDataType=sfix(16)  ParameterScaling=2^0  OutDataType=sfix(16)  OutScaling=2^0  SaturateOnIntegerOverflow=on  OutDataTypeStr=Inherit: Same as input  ParamDataTypeStr=Inherit: Same as input
  sensors : Outport  OutDataType=sfix(16)  OutScaling=2^0
  wires:
  25 msec delay4/1 -> Bus Creator1/5  "accels_cg"
  25 msec delay3/1 -> Bus Creator1/4  "NED_dot"
  25 msec delay2/1 -> Bus Creator1/3  "e"
  25 msec delay1/1 -> Demux1/1
  25 msec delay6/1 -> Bus Creator1/8  "NED_wind"
  Bus Selector1/8 -> 25 msec delay6/1  "<NED_wind>"
  25 msec delay5/1 -> Bus Creator1/7  "u_meas"
  Bus Selector1/7 -> 25 msec delay5/1  "<u_meas>"
  Bus Selector1/6 -> Bus Creator1/6  "<nav_ok>"
  Bus Selector1/5 -> 25 msec delay4/1  "<accels_cg>"
  Bus Selector1/4 -> 25 msec delay3/1  "<NED_dot>"
  Bus Selector1/3 -> 25 msec delay2/1  "<e>"
  Bus Selector1/2 -> 25 msec delay1/1  "<latlonh>"
  Bus Selector1/1 -> 25 msec delay/1  "<pqr>"
  Bus Selector1/9 -> Bus Creator1/9  "<seeker>"
  25 msec delay/1 -> Bus Creator1/1  "pqr"
  Bus Creator/1 -> Bus Selector1/1
  Mux/1 -> Bus Creator1/2  "latlonh"
  Demux1/3 -> Mux/3  "h"
  Demux1/2 -> Mux/2  "lon"
  Demux1/1 -> Mux/1  "lat"
  Bus Creator1/1 -> sensors/1
  Signal Specification/1 -> Bus Creator/7  "u_meas"
  Bus Selector/5 -> Signal Specification/1  "<u_servo>"
  use_wind_meas_sim/1 -> Bus Creator/8  "NED_wind"
  Gain1/1 -> Bus Creator/4  "NED_dot"
  NEh2LLh/1 -> Bus Creator/2  "latlonh"
  pqr/1 -> Bus Creator/1  "pqr"
  NEh_dot/1 -> Gain1/1  "NEh_dot"
  Bus Selector/2 -> NEh_dot/1  "<xdot>"
  quat/1 -> Bus Creator/3  "e"
  initial position/1 -> NEh2LLh/2
  Constant/1 -> Bus Creator/6  "nav_ok"
  NEh/1 -> NEh2LLh/1
  output_bus/1 -> Bus Selector/1
  Bus Selector/6 -> use_wind_meas_sim/1  "<NED_wind>"
  seeker/1 -> Bus Creator/9  "seeker"
  Bus Selector/1 -> quat/1, NEh/1, pqr/1  "<x>"
  Bus Selector/3 -> Bus Creator/5  "<accels_cg>"
  Bus Selector/4 -> Terminator/1  "<dircos>"

== system models/tmp - 1st order sensor model ==
  note: VARIABLE RATE LIMIT SENSOR MODEL
      | (1st order with delay)
  sens_bus : Inport  OutDataType=sfix(16)  OutScaling=2^0
  1st order sensor model : Subsystem
  sens_out : Outport  OutDataType=sfix(16)  OutScaling=2^0
  wires:
  sens_bus/1 -> 1st order sensor model/1(act_bus)
  1st order sensor model/1(u_pos) -> sens_out/1

== system models/tmp - 1st order sensor model with delay ==
  note: VARIABLE RATE LIMIT SENSOR MODEL
      | (1st order with delay)
  sens_bus : Inport  OutDataType=sfix(16)  OutScaling=2^0
  Transport Delay : TransportDelay  DelayTime=SENSOR.delay  InitialOutput=SENSOR.x0
  sens_out : Outport  OutDataType=sfix(16)  OutScaling=2^0
  wires:
  Transport Delay/1 -> sens_out/1
  ? -> Transport Delay/1
  sens_bus/1 -> ?

== system models/gtm-aero/A/C parameters ==
  Engines : Inport  OutDataType=sfix(16)  OutScaling=2^0
  Surfaces : Inport  Port=2  OutDataType=sfix(16)  OutScaling=2^0
  B : Constant  Value=b  OutDataType=sfix(16)  OutScaling=2^0
  Bus Creator4 : BusCreator  Inputs=15
  Bus Selector : BusSelector  OutputSignals=fuel_used
  Bus Selector1 : BusSelector  OutputSignals=GEAR
  Cbar : Constant  Value=Cbar  OutDataType=sfix(16)  OutScaling=2^0
  Demux : Demux  Outputs=6
  Inertia/Mass/CG Shift : Subsystem  mask{DamageModels=DamageModels}
      mask prompts: DamageModels "Array of Damage Cases"
      mask init:
      | Ncases=length(DamageModels);
      | dCGDamage=zeros(Ncases+1,3);   
      | dMassDamage=zeros(Ncases+1,1);
      | dInertiaDamage=zeros(Ncases+1,6);
      | for i=1:Ncases,
      |   if isfield(DamageModels{i},'Mass'),
      |      dInertiaDamage(i+1,:)=DamageModels{i}.Mass.dIxxIyyIzzIxzIyzIxy;
      |      dCGDamage(i+1,:)=DamageModels{i}.Mass.dCG;
      |      dMassDamage(i+1)=DamageModels{i}.Mass.dWeight;
      |   end
      | end
  S : Constant  Value=S  OutDataType=sfix(16)  OutScaling=2^0
  TriggerDamage : Subsystem
  ixxb5 : Constant  Value=engr_pos  OutDataType=sfix(16)  OutScaling=2^0
  ixxb6 : Constant  Value=engl_pos  OutDataType=sfix(16)  OutScaling=2^0
  xCG1 : Constant  Value=ref_cg  OutDataType=sfix(16)  OutScaling=2^0
  AC_parameters : Outport  OutDataType=sfix(16)  OutScaling=2^0
  wires:
  Bus Selector/1 -> Inertia/Mass/CG Shift/2(fuel_used)
  Bus Selector1/1 -> Inertia/Mass/CG Shift/1(gear)
  [DamageCase] -> Inertia/Mass/CG Shift/3(DamageCase)
  [DamageCase] -> Bus Creator4/13  "DamageCase"
  Inertia/Mass/CG Shift/3(CG) -> Bus Creator4/12  "CG"
  Inertia/Mass/CG Shift/2(mass) -> Bus Creator4/11  "mass"
  Demux/6 -> Bus Creator4/10  "Ixy"
  Demux/5 -> Bus Creator4/9  "Iyz"
  Demux/4 -> Bus Creator4/8  "Ixz"
  Demux/3 -> Bus Creator4/7  "Izz"
  Demux/2 -> Bus Creator4/6  "Iyy"
  Demux/1 -> Bus Creator4/5  "Ixx"
  ixxb6/1 -> Bus Creator4/15  "LfEng"
  ixxb5/1 -> Bus Creator4/14  "RtEng"
  xCG1/1 -> Bus Creator4/4  "CP"
  B/1 -> Bus Creator4/3  "B"
  Cbar/1 -> Bus Creator4/2  "Cbar"
  S/1 -> Bus Creator4/1  "S"
  TriggerDamage/1(damagecase) -> [DamageCase]
  Inertia/Mass/CG Shift/1(Inertia) -> Demux/1
  Surfaces/1 -> Bus Selector1/1
  Engines/1 -> Bus Selector/1
  Bus Creator4/1 -> AC_parameters/1

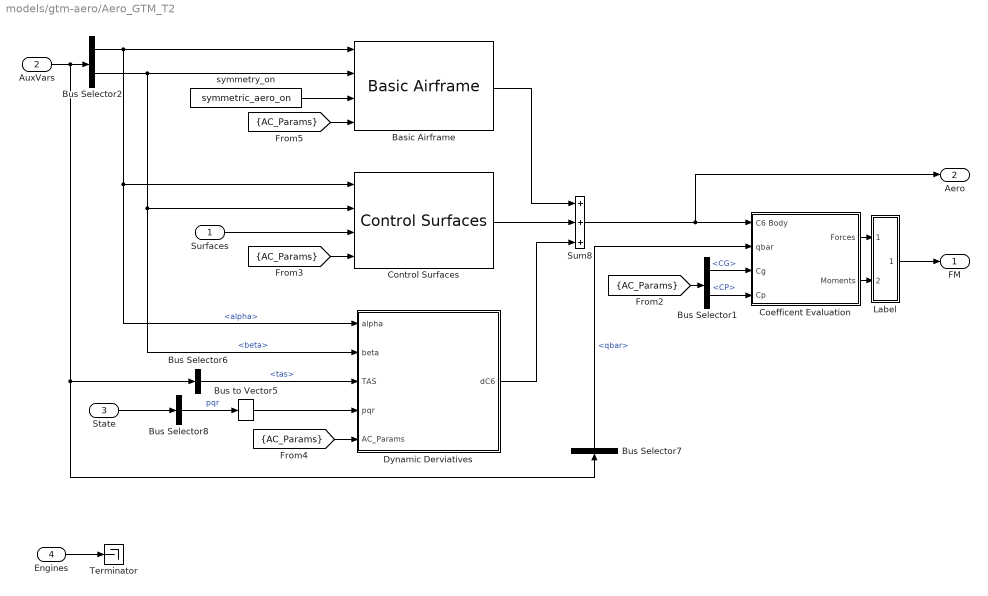
== system models/gtm-aero/Aero_GTM_T2 ==
  Surfaces : Inport  OutDataType=sfix(16)  OutScaling=2^0
  AuxVars : Inport  Port=2  OutDataType=sfix(16)  OutScaling=2^0
  State : Inport  Port=3  OutDataType=sfix(16)  OutScaling=2^0
  Engines : Inport  Port=4  OutDataType=sfix(16)  OutScaling=2^0
  Basic Airframe : GTM_aerolib/Basic Airframe  SystemSampleTime=-1
  Bus Selector1 : BusSelector  OutputSignals=CG,CP
  Bus Selector2 : BusSelector  OutputSignals=alpha,beta
  Bus Selector6 : BusSelector  OutputSignals=tas
  Bus Selector7 : BusSelector  Orientation=up  OutputSignals=qbar
  Bus Selector8 : BusSelector  OutputSignals=pb,qb,rb  OutputAsBus=on
  Bus to Vector5 : BusToVector
  Coefficent Evaluation : Subsystem  AncestorBlock=aeroutilslib/Coefficent Evaluation  mask{b=b, cbar=Cbar, Sref=S}
      mask prompts: b "Reference Span (b)"; cbar "Reference Chord (cbar)"; Sref "Reference Area (Sref)"
      mask help:
      | Calulates the Force and Moments due to aerodynamic loads from vector of body axes aerodynamic coefficients:
      |    C6body = [Cx Cy Cz Cl Cm Cn].
      | Also requires dynamic pressure, cg/cp locations and reference lengths/area.
  Control Surfaces : GTM_aerolib/Control Surfaces  SystemSampleTime=-1
  Dynamic Derviatives : Subsystem  AncestorBlock=GTM_aerolib/Dynamic Derviatives
  Label : Subsystem
  Sum8 : Sum  Inputs=+++  OutDataType=sfix(16)  OutScaling=2^0  SaturateOnIntegerOverflow=on  InputSameDT=on  OutDataTypeStr=Inherit: Same as first input
  Terminator : Terminator
  symmetry_on : Constant  Value=symmetric_aero_on  OutDataType=sfix(16)  OutScaling=2^0
  FM : Outport  OutDataType=sfix(16)  OutScaling=2^0
  Aero : Outport  Port=2  OutDataType=sfix(16)  OutScaling=2^0
  wires:
  [AC_Params] -> Dynamic Derviatives/5(AC_Params)
  Bus to Vector5/1 -> Dynamic Derviatives/4(pqr)
  Bus Selector6/1 -> Dynamic Derviatives/3(TAS)  "<tas>"
  [AC_Params] -> Control Surfaces/4
  [AC_Params] -> Basic Airframe/4
  Bus Selector8/1 -> Bus to Vector5/1  "pqr"
  Engines/1 -> Terminator/1
  Basic Airframe/1 -> Sum8/1
  Control Surfaces/1 -> Sum8/2
  Dynamic Derviatives/1(dC6) -> Sum8/3
  State/1 -> Bus Selector8/1
  Bus Selector2/2 -> Basic Airframe/2, Dynamic Derviatives/2(beta), Control Surfaces/2  "<beta>"
  Bus Selector2/1 -> Basic Airframe/1, Dynamic Derviatives/1(alpha), Control Surfaces/1  "<alpha>"
  AuxVars/1 -> Bus Selector2/1, Bus Selector6/1, Bus Selector7/1
  Label/1(O) -> FM/1
  Bus Selector7/1 -> Coefficent Evaluation/2(qbar)  "<qbar>"
  Sum8/1 -> Aero/1, Coefficent Evaluation/1(C6 Body)
  Coefficent Evaluation/1(Forces) -> Label/1(If)
  Coefficent Evaluation/2(Moments) -> Label/2(Im)
  Bus Selector1/1 -> Coefficent Evaluation/3(Cg)  "<CG>"
  [AC_Params] -> Bus Selector1/1
  Bus Selector1/2 -> Coefficent Evaluation/4(Cp)  "<CP>"
  symmetry_on/1 -> Basic Airframe/3
  Surfaces/1 -> Control Surfaces/3

== system models/gtm-aero/AuxVars_Reduced ==
  pqr : Inport  OutDataType=sfix(16)  OutScaling=2^0
  aero_env : Inport  Port=2  OutDataType=sfix(16)  OutScaling=2^0
  P : Inport  Port=3  OutDataType=sfix(16)  OutScaling=2^0
  T : Inport  Port=4  OutDataType=sfix(16)  OutScaling=2^0
  Bus Creator : BusCreator  Inputs=6
  Bus Creator1 : BusCreator  Inputs=3
  Bus Selector : BusSelector  OutputSignals=qbar,alpha,beta,vel
  Demux : Demux  Outputs=3
  Gain : Gain  Gain=1/atmos.alt_T0  ParameterDataType=sfix(16)  ParameterScaling=2^0  OutDataType=sfix(16)  OutScaling=2^0
  Gain1 : Gain  Gain=1/atmos.alt_P0  ParameterDataType=sfix(16)  ParameterScaling=2^0  OutDataType=sfix(16)  OutScaling=2^0
  Gain2 : Gain  Gain=180/pi  ParameterDataType=sfix(16)  ParameterScaling=2^0  OutDataType=sfix(16)  OutScaling=2^0
  Gain3 : Gain  Gain=180/pi  ParameterDataType=sfix(16)  ParameterScaling=2^0  OutDataType=sfix(16)  OutScaling=2^0
  Gain5 : Gain  Gain=1/1.689  ParameterDataType=sfix(16)  ParameterScaling=2^0  OutDataType=sfix(16)  OutScaling=2^0
  AuxVars : Outport  OutDataType=sfix(16)  OutScaling=2^0
  State : Outport  Port=2  OutDataType=sfix(16)  OutScaling=2^0
  wires:
  Gain5/1 -> Bus Creator/4  "tas"
  Bus Creator/1 -> AuxVars/1
  Gain/1 -> Bus Creator/6  "tratio"
  Bus Selector/4 -> Gain5/1  "<vel>"
  Bus Selector/3 -> Gain3/1  "<beta>"
  Bus Selector/2 -> Gain2/1  "<alpha>"
  Bus Selector/1 -> Bus Creator/1  "<qbar>"
  Bus Creator1/1 -> State/1
  Demux/3 -> Bus Creator1/3  "rb"
  Demux/2 -> Bus Creator1/2  "qb"
  Demux/1 -> Bus Creator1/1  "pb"
  pqr/1 -> Demux/1
  Gain1/1 -> Bus Creator/5  "pratio"
  T/1 -> Gain/1
  P/1 -> Gain1/1
  aero_env/1 -> Bus Selector/1
  Gain2/1 -> Bus Creator/2  "alpha"
  Gain3/1 -> Bus Creator/3  "beta"

== system models/gtm-aero/aero surf ganging ==
  u : Inport  OutDataType=sfix(16)  OutScaling=2^0
  Actuator_GTM_T2 (modified) : Subsystem  AncestorBlock=actuator_T2_lib/GTM_T2
  Input Generator (modified) : Subsystem  AncestorBlock=UserContent_lib/Input Generator
  cmds : Outport  OutDataType=sfix(16)  OutScaling=2^0
  wires:
  u/1 -> Input Generator (modified)/1(Feedback)
  Input Generator (modified)/1(cmds) -> Actuator_GTM_T2 (modified)/1(cmds)
  Actuator_GTM_T2 (modified)/1(Surface Pos) -> cmds/1
  Input Generator (modified)/2(cmd_stab) -> Actuator_GTM_T2 (modified)/2(cmd_stab)

== system models/gtm-aero (for V0905)/A/C parameters ==
  Engines : Inport  OutDataType=sfix(16)  OutScaling=2^0
  Surfaces : Inport  Port=2  OutDataType=sfix(16)  OutScaling=2^0
  B : Constant  Value=b  OutDataType=sfix(16)  OutScaling=2^0
  Bus Creator4 : BusCreator  Inputs=15
  Bus Selector : BusSelector  OutputSignals=fuel_used
  Bus Selector1 : BusSelector  OutputSignals=GEAR
  Cbar : Constant  Value=Cbar  OutDataType=sfix(16)  OutScaling=2^0
  Demux : Demux  Outputs=6
  Inertia/Mass/CG Shift : Subsystem  mask{DamageModels=DamageModels}
      mask prompts: DamageModels "Array of Damage Cases"
      mask init: same as models/gtm-aero/A/C parameters/Inertia/Mass/CG Shift
  S : Constant  Value=S  OutDataType=sfix(16)  OutScaling=2^0
  TriggerDamage : Subsystem
  ixxb5 : Constant  Value=engr_pos  OutDataType=sfix(16)  OutScaling=2^0
  ixxb6 : Constant  Value=engl_pos  OutDataType=sfix(16)  OutScaling=2^0
  xCG1 : Constant  Value=ref_cg  OutDataType=sfix(16)  OutScaling=2^0
  AC_parameters : Outport  OutDataType=sfix(16)  OutScaling=2^0
  wires:
  Bus Creator4/1 -> AC_parameters/1
  Engines/1 -> Bus Selector/1
  Surfaces/1 -> Bus Selector1/1
  Inertia/Mass/CG Shift/1(Inertia) -> Demux/1
  TriggerDamage/1(damagecase) -> [DamageCase]
  S/1 -> Bus Creator4/1  "S"
  Cbar/1 -> Bus Creator4/2  "Cbar"
  B/1 -> Bus Creator4/3  "B"
  xCG1/1 -> Bus Creator4/4  "CP"
  ixxb5/1 -> Bus Creator4/14  "RtEng"
  ixxb6/1 -> Bus Creator4/15  "LfEng"
  Demux/1 -> Bus Creator4/5  "Ixx"
  Demux/2 -> Bus Creator4/6  "Iyy"
  Demux/3 -> Bus Creator4/7  "Izz"
  Demux/4 -> Bus Creator4/8  "Ixz"
  Demux/5 -> Bus Creator4/9  "Iyz"
  Demux/6 -> Bus Creator4/10  "Ixy"
  Inertia/Mass/CG Shift/2(mass) -> Bus Creator4/11  "mass"
  Inertia/Mass/CG Shift/3(CG) -> Bus Creator4/12  "CG"
  [DamageCase] -> Bus Creator4/13  "DamageCase"
  [DamageCase] -> Inertia/Mass/CG Shift/3(DamageCase)
  Bus Selector1/1 -> Inertia/Mass/CG Shift/1(gear)
  Bus Selector/1 -> Inertia/Mass/CG Shift/2(fuel_used)

== system models/gtm-aero (for V0905)/Aero_GTM_T2 ==
  Surfaces : Inport  OutDataType=sfix(16)  OutScaling=2^0
  AuxVars : Inport  Port=2  OutDataType=sfix(16)  OutScaling=2^0
  State : Inport  Port=3  OutDataType=sfix(16)  OutScaling=2^0
  Engines : Inport  Port=4  OutDataType=sfix(16)  OutScaling=2^0
  Basic Airframe : GTM_aerolib/Basic Airframe  SystemSampleTime=-1
  Bus Selector1 : BusSelector  OutputSignals=CG,CP
  Bus Selector2 : BusSelector  OutputSignals=alpha,beta
  Bus Selector6 : BusSelector  OutputSignals=tas
  Bus Selector7 : BusSelector  Orientation=up  OutputSignals=qbar
  Bus Selector8 : BusSelector  OutputSignals=pb,qb,rb  OutputAsBus=on
  Bus to Vector5 : BusToVector
  Coefficent Evaluation : Subsystem  AncestorBlock=aeroutilslib/Coefficent Evaluation  mask{b=b, cbar=Cbar, Sref=S}
      mask prompts: b "Reference Span (b)"; cbar "Reference Chord (cbar)"; Sref "Reference Area (Sref)"
      mask help:
      | Calulates the Force and Moments due to aerodynamic loads from vector of body axes aerodynamic coefficients:
      |    C6body = [Cx Cy Cz Cl Cm Cn].
      | Also requires dynamic pressure, cg/cp locations and reference lengths/area.
  Control Surfaces : GTM_aerolib/Control Surfaces  SystemSampleTime=-1
  Dynamic Derviatives : Subsystem  AncestorBlock=GTM_aerolib/Dynamic Derviatives
  Label : Subsystem
  Sum8 : Sum  Inputs=+++  OutDataType=sfix(16)  OutScaling=2^0  SaturateOnIntegerOverflow=on  InputSameDT=on  OutDataTypeStr=Inherit: Same as first input
  Terminator : Terminator
  symmetry_on : Constant  Value=symmetric_aero_on  OutDataType=sfix(16)  OutScaling=2^0
  FM : Outport  OutDataType=sfix(16)  OutScaling=2^0
  Aero : Outport  Port=2  OutDataType=sfix(16)  OutScaling=2^0
  wires:
  Surfaces/1 -> Control Surfaces/3
  symmetry_on/1 -> Basic Airframe/3
  Bus Selector1/2 -> Coefficent Evaluation/4(Cp)  "<CP>"
  [AC_Params] -> Bus Selector1/1
  Bus Selector1/1 -> Coefficent Evaluation/3(Cg)  "<CG>"
  Coefficent Evaluation/2(Moments) -> Label/2(Im)
  Coefficent Evaluation/1(Forces) -> Label/1(If)
  Sum8/1 -> Coefficent Evaluation/1(C6 Body), Aero/1
  Bus Selector7/1 -> Coefficent Evaluation/2(qbar)  "<qbar>"
  Label/1(O) -> FM/1
  AuxVars/1 -> Bus Selector7/1, Bus Selector6/1, Bus Selector2/1
  Bus Selector2/1 -> Control Surfaces/1, Dynamic Derviatives/1(alpha), Basic Airframe/1  "<alpha>"
  Bus Selector2/2 -> Control Surfaces/2, Dynamic Derviatives/2(beta), Basic Airframe/2  "<beta>"
  State/1 -> Bus Selector8/1
  Dynamic Derviatives/1(dC6) -> Sum8/3
  Control Surfaces/1 -> Sum8/2
  Basic Airframe/1 -> Sum8/1
  Engines/1 -> Terminator/1
  Bus Selector8/1 -> Bus to Vector5/1  "pqr"
  [AC_Params] -> Basic Airframe/4
  [AC_Params] -> Control Surfaces/4
  Bus Selector6/1 -> Dynamic Derviatives/3(TAS)  "<tas>"
  Bus to Vector5/1 -> Dynamic Derviatives/4(pqr)
  [AC_Params] -> Dynamic Derviatives/5(AC_Params)
